simulink model "AirFlow"  (R2015a)
settings: Solver=ode45  StartTime=0.0  StopTime=10.0  RelTol=1e-3
libraries: simulink x1
settings Model: Creator=laragoxhaj  LastModifiedBy=laragoxhaj

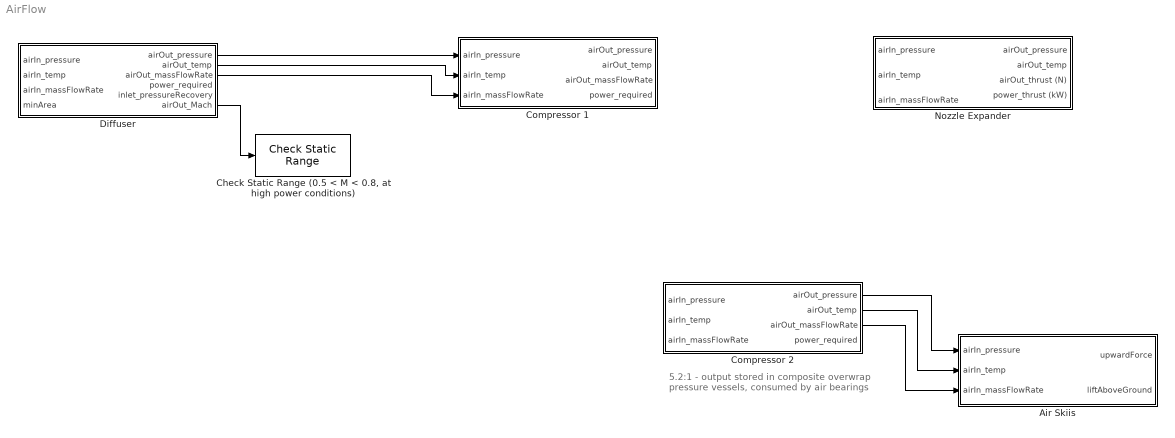
== system AirFlow ==
  note: 5.2:1 - output stored in composite overwrap
      | pressure vessels, consumed by air bearings
  Air Skiis : Subsystem
  "Check Static Range (0.5 < M < 0.8, at high power conditions)" : simulink/Model Verification/Check  Static Range  Description=0.5 <= u <= 0.8  max=0.8  max_included=on  min=0.5  min_included=on  enabled=on  stopWhenAssertionFail=on  export=off  icon=graphic
  Compressor 1 : Subsystem
  Compressor 2 : Subsystem
  Diffuser : Subsystem
  Nozzle Expander : Subsystem
  wires:
  Diffuser/1(airOut_pressure) -> Compressor 1/1(airIn_pressure)
  Diffuser/2(airOut_temp) -> Compressor 1/2(airIn_temp)
  Diffuser/3(airOut_massFlowRate) -> Compressor 1/3(airIn_massFlowRate)
  Diffuser/6(airOut_Mach) -> "Check Static Range (0.5 < M < 0.8, at high power conditions)"/1
  Compressor 2/1(airOut_pressure) -> Air Skiis/1(airIn_pressure)
  Compressor 2/2(airOut_temp) -> Air Skiis/2(airIn_temp)
  Compressor 2/3(airOut_massFlowRate) -> Air Skiis/3(airIn_massFlowRate)

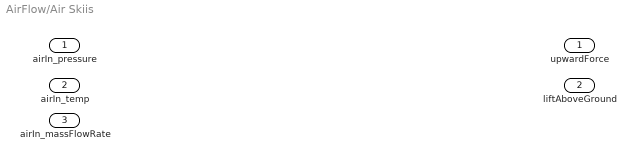
== system AirFlow/Air Skiis ==
  airIn_pressure : Inport
  airIn_temp : Inport  Port=2
  airIn_massFlowRate : Inport  Port=3
  upwardForce : Outport
  liftAboveGround : Outport  Port=2

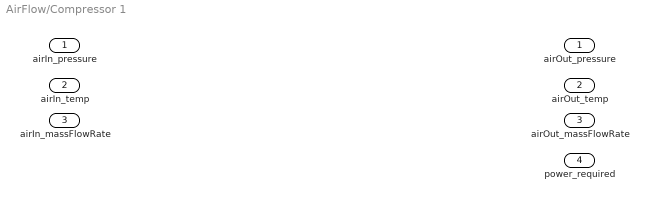
== system AirFlow/Compressor 1 ==
  airIn_pressure : Inport
  airIn_temp : Inport  Port=2
  airIn_massFlowRate : Inport  Port=3
  airOut_pressure : Outport
  airOut_temp : Outport  Port=2
  airOut_massFlowRate : Outport  Port=3
  power_required : Outport  Port=4

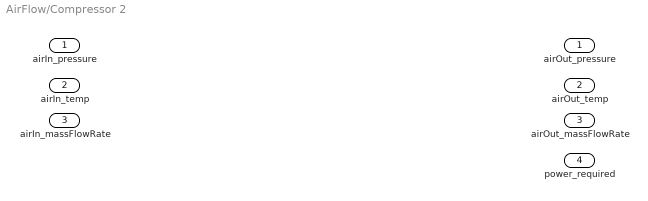
== system AirFlow/Compressor 2 ==
  airIn_pressure : Inport
  airIn_temp : Inport  Port=2
  airIn_massFlowRate : Inport  Port=3
  airOut_pressure : Outport
  airOut_temp : Outport  Port=2
  airOut_massFlowRate : Outport  Port=3
  power_required : Outport  Port=4

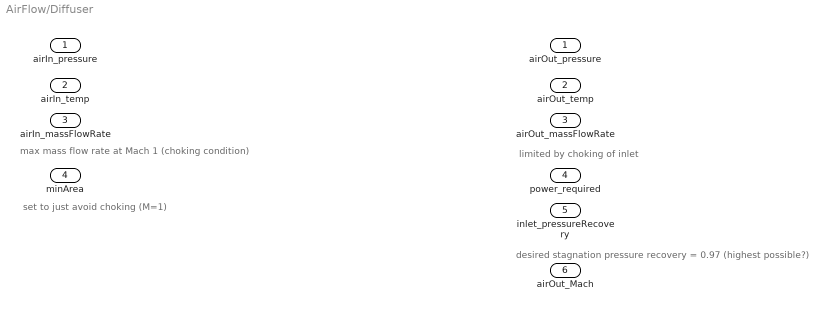
== system AirFlow/Diffuser ==
  note: set to just avoid choking (M=1)
  note: desired stagnation pressure recovery = 0.97 (highest possible?)
  note: limited by choking of inlet
  note: max mass flow rate at Mach 1 (choking condition)
  airIn_pressure : Inport
  airIn_temp : Inport  Port=2
  airIn_massFlowRate : Inport  Port=3
  minArea : Inport  Port=4
  airOut_pressure : Outport
  airOut_temp : Outport  Port=2
  airOut_massFlowRate : Outport  Port=3
  power_required : Outport  Port=4
  inlet_pressureRecovery : Outport  Port=5
  airOut_Mach : Outport  Port=6

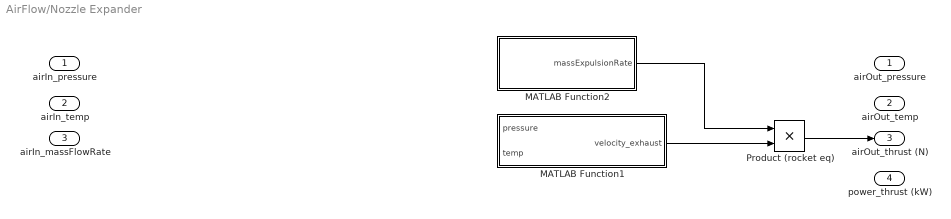
== system AirFlow/Nozzle Expander ==
  airIn_pressure : Inport
  airIn_temp : Inport  Port=2
  airIn_massFlowRate : Inport  Port=3
  MATLAB Function1 : MATLAB Function  TreatAsAtomicUnit=on
  MATLAB Function2 : MATLAB Function  TreatAsAtomicUnit=on
  Product (rocket eq) : Product
  airOut_pressure : Outport
  airOut_temp : Outport  Port=2
  airOut_thrust (N) : Outport  Port=3
  power_thrust (kW) : Outport  Port=4
  wires:
  Product (rocket eq)/1 -> airOut_thrust (N)/1
  MATLAB Function2/1(massExpulsionRate) -> Product (rocket eq)/1
  MATLAB Function1/1(velocity_exhaust) -> Product (rocket eq)/2

== matlab function AirFlow/Nozzle Expander/MATLAB Function1 ==
  data: pressure input; velocity_exhaust output; temp input
% m/s
function velocity_exhaust = fcn(pressure, temp)
velocity_exhaust = sqrt(2 * pressure * temp);

== matlab function AirFlow/Nozzle Expander/MATLAB Function2 ==
  data: massExpulsionRate output
% N
% rocket equation
function massExpulsionRate = massExpulse()
massExpulsionRate = 0;
